simulink model "sim2"  (R2017b)
settings: Solver=VariableStepAuto  StartTime=0.0  StopTime=10.0  RelTol=1e-3
settings Model: Creator=Administrator  LastModifiedBy=Administrator

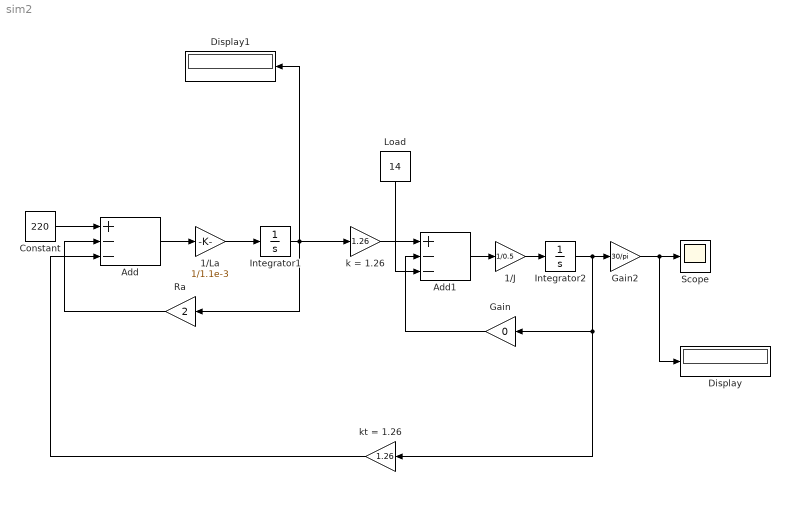
== system sim2 ==
  "1/J " : Gain  Gain=1/0.5
  "1/La " : Gain  Gain=1/1.1e-3
  Add : Sum  Inputs=+--
  Add1 : Sum  Inputs=+--
  Constant : Constant  Value=220
  Display : Display
  Display1 : Display
  Gain : Gain  Gain=0
  Gain2 : Gain  Gain=30/pi
  Integrator1 : Integrator
  Integrator2 : Integrator
  Load : Constant  Value=14
  "Ra " : Gain  Gain=2
  Scope : Scope
  k = 1.26 : Gain  Gain=1.26
  kt = 1.26 : Gain  Gain=1.26
  wires:
  Add/1 -> "1/La "/1
  "1/La "/1 -> Integrator1/1
  "1/J "/1 -> Integrator2/1
  Load/1 -> Add1/3
  Constant/1 -> Add/1
  Integrator1/1 -> Display1/1, "Ra "/1, k = 1.26/1
  "Ra "/1 -> Add/2
  k = 1.26/1 -> Add1/1
  Add1/1 -> "1/J "/1
  Integrator2/1 -> Gain2/1, Gain/1, kt = 1.26/1
  kt = 1.26/1 -> Add/3
  Gain/1 -> Add1/2
  Gain2/1 -> Display/1, Scope/1
